simulink library "carnot"  (R2018b)
settings: Solver=VariableStepAuto  StartTime=0.0  StopTime=10.0  RelTol=1e-3
undefined symbols (not defined in the file or in its folder): A, A_earth, acol, Acol, ActPower1, ActPower2, ActPower3, Ad, Ad0, Ar, Au, Au0, Azimuth_Angle, B, Bd, Bd0, Br, Bu, Bu0, C, c1, c2, c3, c33, c4, c5, c6, CarnotCallbacks_Density, CarnotCallbacks_Enthalpy, CarnotCallbacks_Enthalpy2Temperature, CarnotCallbacks_Entropy, CarnotCallbacks_Evaporation_Enthalpy, CarnotCallbacks_GlobalMessageLevel, CarnotCallbacks_Grashof, CarnotCallbacks_Heat_Capacity, CarnotCallbacks_Kinematic_Viscosity, CarnotCallbacks_PMV_PPD, CarnotCallbacks_Prandtl, CarnotCallbacks_Saturation_Property, CarnotCallbacks_Saturation_Temperature, CarnotCallbacks_Saturation_Value_Water, CarnotCallbacks_Specific_Volume, CarnotCallbacks_Thermal_Conductivity, CarnotCallbacks_Vapour_Content, CarnotCallbacks_Vapour_Pressure, Cd, Cdl, Cr, Cu, Davies, Dd, DE_TRY2010_04_averageYear, delta_grd, density, DiameterLastPiece, dl, DPConstant, DPLinear, DPQuadratic, Dr ... (+59)
libraries: $bdroot x429, simulink x36, simulink_extras x12
(part 2 of 22)

== system carnot/Hydraulics ==
  Fan_Const : Subsystem  mask(Fan constant){Vdotmax=1000, dia=0.5, p0=101300, mix=0.01, Tini=20, UA=3, mcp=1000, e0=10, e1=10, e2=-1}
      mask prompts: Vdotmax "Vdotmax : volume flowrate in m³/h"; dia "diameter at in- and outlet [m]"; p0 "air pressure in Pa"; mix "kg of water per kg of dry air"; Tini "ambient and start temperature in °C"; UA "Thermal loss coefficient to ambient in W/K"; mcp "mcp: thermal capacity of the node in J/K"; e0 "e0: constant coefficient in W"; e1 "e1: linear coefficient in W*s/kg"; e2 "e2: quadratic coefficient in W*(s/kg)²"
      mask help:
      | Model of a fan for air ventilation systems. Volume flowrate is constant according to the parameter Vdotmax and the control signal:
      | Vdot = Vdotmax * Ctrl
      | Keep in mind that the flowrate in the THB is the massflowrate in kg/s whereas the parameters of the fan have different units.
      | mdot = Vdot/3600 * density(Tamb, air_pressure, FluidAir, kgH2O/kgAir)
      | Use the option "thermal node" if you want the pump to have thermal capacity and losses to ambient (or if you want to break an algebraic loop in the temperature signal).
      | Electric power is calculated Pel = e0 + e1*mdot + e2*mdot^2
      mask Help: web(fullfile(path_carnot('help'),'Fan_Const.html'),'-helpbrowser')
      mask TypeOptions dia: Pump_Const/dia
      mask TypeOptions mix: Pump_Const/mix
      mask TypeOptions Tini: Pump_Const/Tini
      mask TypeOptions UA: Pump_Const/UA
      mask TypeOptions mcp: Pump_Const/mcp
      mask TypeOptions e0: Pump_Const/e0
      mask TypeOptions e1: Pump_Const/e1
      mask TypeOptions e2: Pump_Const/e2
      mask DialogControl ParameterTabVar0 Prompt: Hydraulic
      mask DialogControl Container7 Prompt: Initial Values
      mask DialogControl ParameterTabVar012 Prompt: Thermal
      mask DialogControl ParameterTabVar01 Prompt: Electric
      mask Display:
      | plot(-40,-20,130,100, ...
      |     [0,0,10,30,50,70,80,80,70,50,30,10,0],[50,30,10,0,0,10,30,50,70,80,80,70,50], ...
      |     [80,10],[50,70], ...
      |     [80,10],[30,10])
  Flow_Diverter : Subsystem  mask(flow diverter, fixed rate){}
      mask help:
      | The block diverts an incoming massflow according to:
      | mdot1 = mdot * fdiv
      | mdot2 = mdot * (1-fdiv)
      | fdiv is limited to the range [0..1]
      mask Help: web(fullfile(path_carnot('help'),'Flow_Diverter.html'),'-helpbrowser')
      mask Display: plot(0,-5,120,65,[20 45 20 20],[20 30 40 20],[45 70 70 45],[30 20 40 30],[45 35 55 45],[30 10 10 30])
  Flow_Mixer : Subsystem  mask(flow mixer){}
      mask help:
      | Mixes two massflows. The new temperature is calculated by an energy balance. The output f_div may be fed back to the corresponding flow diverter upwards in flowdirection.
      | This model uses a Memory block to break an algebraic loop. Avoid using the variable-step solver ode15s or ode113 (see block help for details).
      mask Help: web(fullfile(path_carnot('help'),'Flow_Mixer.html'),'-helpbrowser')
      mask Display: plot(-25,-5,95,65,[20 45 20 20],[20 30 40 20],[45 70 70 45],[30 20 40 30],[45 35 55 45],[30 10 10 30])
  Flow_Mixer_Thermostatic : Subsystem  mask(thermostatic flow mixer){t=10}
      mask prompts: t "time constant for valve [s]"
      mask help:
      | The thermostatic flow mixer mixes cold and hot fluid to set a desired temperature and calculates the pressure drop.
      | Use together with flow_diverter_fixed_rate.
      mask init:
      | if t < 0.01
      |     t = 0.01;
      |     disp('Flow mixer thermostatic: time constant set to minimum value 0.01')
      | end
      | t1 = 1/t;
      mask Help: web(fullfile(path_carnot('help'),'Flow_Mixer.html'),'-helpbrowser')
      mask Display: plot(10,0,100,100,[40,60,60,40,40],[60,40,60,40,60],[44,50,56,44],[66,50,66,66],[50,50],[30,50],[56,44],[25,25],[50,50],[10,25])
  Mixing_Valve : Subsystem  mask(Mixing Valve){Art_A=equal percentage, Art_B=linear, kvs=1.6, psi_0=0.01, dt_V=30}
      mask prompts: Art_A "Valve characteristic A->AB"; Art_B "Valve characteristic B->AB"; kvs "Kvs: flow coefficient of the open valve in m³/h"; psi_0 "Psi_0: relative flow coefficient Kv/Kvs of the closed valve"; dt_V "Valve running time in s"
      mask help:
      | Mixes two massflows and calculates the pressure drop of the branches. The new temperature is calculated by an energy balance. The output f_div may be fed back to the corresponding flow diverter upwards in flowdirection.
      | This model uses a Memory block to break an algebraic loop. Avoid using the variable-step solver ode15s or ode113 (see block help for details).
      mask Help: web(fullfile(path_carnot('help'),'Mixing_Valve.html'),'-helpbrowser')
      mask TypeOptions Art_A: Valve_A/vtyp
      mask TypeOptions Art_B: Valve_B/vtyp
      mask TypeOptions kvs: Valve_A/kvs | Valve_B/kvs
      mask TypeOptions psi_0: Valve_A/psi_0 | Valve_B/psi_0
      mask TypeOptions dt_V: Valve_A/dt_V | Valve_B/dt_V
      mask Display:
      | plot(-20,-5,110,90,...
      |     [20 50 20 20],[20 30 40 20],...
      |     [50 80 80 50],[30 20 40 30],...
      |     [50 40 60 50],[30 10 10 30],...
      |     [50,50],[45,30],...
      |     [40,30,30,40,60,70,70,60,40],[45,50,60,65,65,60,50,45,45],...
      |     [60,60,50,40,40],[50,60,55,60,50])
  Pipe : Subsystem  mask(pipe){dia=0.02, len=10, hgt=5, uloss=100/20/10, cond=0, cwall=1000, t0=20, lin=100/0.2, qua=100/0.2^2, nodes=10}
      mask prompts: dia "diameter [m]"; len "length of pipe [m]"; hgt "static height [m], positive for outlet above"; uloss "heat losses per length [W/(m*K)]"; cond "effective conductivity in axial direction [W/(m*K)]"; cwall "capacity of pipewall per length in [J/(m*K)]"; t0 "initial temperature [degree Celsius]"; lin "pressure drop linear in massflow [Pa*s/kg]"; qua "pressure drop quadratic in massflow [Pa*s²/kg²]"; nodes "number of nodes"
      mask help:
      | Multinode pipe with capacity and simlified pressure drop calculation. The pressure drop is a quadratic function of the massflow. The dependance of the quadratic term on the Reynolds number is neglected. The flow is calculated by the upwind scheme heat conduction between nodes by central differences (Patankar 1980).
      | heat loss: ul = 2*Conductivity*pi*d_in*Length/Length/(d_in*ln(d_out/d_in))
      | The pressure change due to static height can usually be neglected for closes loop pumped systems.
      mask init:
      | if dia < 0.001
      |     dia = 0.001;
      |     disp('Warning in Pipe: diameter set to minimum value 0.001 m')
      | end
      | if len < 0.001
      |     len = 0.001;
      |     disp('Warning in Pipe: length set to minimum value 0.001 m')
      | end
      | if cwall < 0.001
      |     cwall = 0.001;
      |     disp('Warning in Pipe: heat capacity of the wall set to minimum value 0.001 m')
      | end
      | if nodes < 1
      |     nodes = 1;
      |     disp('Warning in Pipe: number of nodes set to minimum 1')
      | end
      mask Help: web(fullfile(path_carnot('help'),'Pipe.html'),'-helpbrowser')
      mask DialogControl ParameterTabVar0 Prompt: Geometry
      mask DialogControl ParameterTabVar01 Prompt: Thermal
      mask DialogControl ParameterTabVar012 Prompt: Hydraulic
      mask DialogControl ParameterTabVar0123 Prompt: Calculation
      mask Display: plot(0,0,100,100,[24,27,27,24,75,80,80,75,24,20,20,24],[60,53,46,40,40,46,55,60,60,53,46,40])
  Pipe_BiFlow : Subsystem  mask(Pipe Biflow){t0=20, hgt=1273.2395, stgtype=1, tini=[20 20 20 20 20 20 20 20 20 20], mpts=[1 2 3 4 5 6 7 8 9 10], PathName=fullfile(path_carnot('libsl'),'Hydraulics','Pipe_BiFlow','parameter_set'), FileName='PipeBF_set1.mat', userPath=off, userParam=off, uwall=1, ubot=0, utop=0, axcond=1, volume=10, dia=0.1, standing=standing cylinder, nodes=10, mpoints=10, pipe1inlet=1, pipe1outlet=0, pipe1dia=0.1, pipe2inlet=0, pipe2outlet=1, pipe2dia=0.1}
      mask prompts: t0 "Initial temperature (vector or scalar) in °C"; hgt "Length of pipe in m"; stgtype "Storage Type (0..5)"; tini "Start temperatures of nodes in °C"; mpts "Index to measured nodes"; PathName "Path"; FileName "Parameter set"; userPath "Edit path and name of parameter set"; userParam "User defined parameters"; uwall "Heat transfer coefficient to ambient [W/m²K]"; ubot "Heat transfer coefficient to ambient bottom [W/m²K]"; utop "Heat transfer coefficient to ambient top [W/m²K]"; axcond "Effective thermal conductivity [W/m/K]"; volume "Volume [m³]"; dia "Diameter [m]"; standing "Position"; nodes "Number of nodes"; mpoints "Number of node temperatures (for display)"; pipe1inlet "relative height of inlet, range from 0 (= bottom) to 1 (= top)"; pipe1outlet "relative height of outlet, range from 0 (= bottom) to 1 (= top)"; pipe1dia "Diameter of connection in m"; pipe2inlet "relative height of inlet, range from 0 (= bottom) to 1 (= top)"; pipe2outlet "relative height of outlet, range from 0 (= bottom) to 1 (= top)"; pipe2dia "Diameter of connection in m"
      mask help: Pipe model for flow in both directions. The model is based on a buffer storage tank but has no calculation for inversed thermocline.
      mask init:
      | [ok, param] = CarnotCallbacks_PipeBiflow('SetParam',1,gcbh,PathName,FileName);
      mask Help: web(fullfile(path_carnot('help'),'PipeBilfow.html'),'-helpbrowser')
      mask TypeOptions hgt: Pipe_Connection_1/hgt | Pipe_Connection_2/hgt
      mask TypeOptions stgtype: CreateSdat/stgtype
      mask TypeOptions tini: sfun_storageTnodes/tini
      mask TypeOptions mpts: select_T/Indices
      mask Callback userPath: [ok, param] = CarnotCallbacks_StorageConf('UserEdit',1,gcbh);
      mask Callback userParam: [ok, param] = CarnotCallbacks_StorageConf('UserEdit',1,gcbh);
      mask TypeOptions uwall: sfun_storageTnodes/uloss
      mask TypeOptions ubot: sfun_storageTnodes/ubot
      mask TypeOptions utop: sfun_storageTnodes/utop
      mask TypeOptions axcond: sfun_storageTnodes/cond
      mask TypeOptions volume: sfun_storageTnodes/volume | CreateSdat/volume
      mask TypeOptions dia: sfun_storageTnodes/dia | Pipe_Connection_1/dstg | Pipe_Connection_2/dstg
      mask TypeOptions standing: sfun_storageTnodes/standing
      mask TypeOptions nodes: sfun_storageTnodes/nodes | select_T/InputPortWidth | HX_EN12977_1/nodes | HX_EN12977_2/nodes | HX_EN12977_3/nodes | Pipe_Connection_1/nodes | Pipe_Connection_2/nodes | Pipe_Connection_3/nodes
      mask TypeOptions pipe1inlet: Pipe_Connection_1/h_in
      mask TypeOptions pipe1outlet: Pipe_Connection_1/h_out
      mask TypeOptions pipe1dia: Pipe_Connection_1/dpipe
      mask TypeOptions pipe2inlet: Pipe_Connection_2/h_in
      mask TypeOptions pipe2outlet: Pipe_Connection_2/h_out
      mask TypeOptions pipe2dia: Pipe_Connection_2/dpipe
      mask DialogControl Container14 Prompt: Infos
      mask DialogControl ParameterGroupVar Prompt: Picking a parameter set
      mask DialogControl Control3 Prompt: Carnot public data
      mask DialogControl Control3 Callback: [ok, file] = CarnotCallbacks_PipeBiflow('GetFilename',1,gcbh,'public');
      mask DialogControl Control4 Prompt: Carnot internal data
      mask DialogControl Control4 Callback: [ok, file] = CarnotCallbacks_PipeBiflow('GetFilename',1,gcbh,'internal');
      mask DialogControl Control2 Prompt: Selected path
      mask DialogControl Control2 Callback: [ok, file] = CarnotCallbacks_PipeBiflow('GetFilename',1,gcbh,'selected');
      mask DialogControl Container4 Prompt: Parameter values
      mask DialogControl Container6 Prompt: Pipe
      mask DialogControl Container8 Prompt: Connections
      mask DialogControl Container9 Prompt: Inlet 1
      mask DialogControl Container12 Prompt: Inlet 2
      mask DialogControl Control6 Prompt: Save in Carnot internal data
      mask DialogControl Control6 Callback: [ok, param] = CarnotCallbacks_PipeBiflow('SaveFilename',1,gcbh,'internal','PipeBF');
      mask DialogControl Control5 Prompt: Save in selected path
      mask DialogControl Control5 Callback: [ok, param] = CarnotCallbacks_PipeBiflow('SaveFilename',1,gcbh,'selected','PipeBF');
      mask Display:
      | % user defined picture file
      | picfile = fullfile(path_carnot('intlibsl'), 'Hydraulics','Pipe_Biflow', ...
      |     'parameter_set', 'Pipe_Biflow.jpg');
      | 
      | % show internal picture if defined
      | pic = false;
      | if  ~BlockIsInCarnotLibrary       % if not located in library
      |     if exist(picfile, 'file')
      |         image(imread(picfile), [0.25, 0, 0.45, 1])
      |         set_param(gcb, 'BackgroundColor', 'White')
      |         pic = true;
      |     end
      | end
      | 
      | % show public picture
      | if ~pic
      |     set_param(gcb, 'BackgroundColor', 'Red')
      |     plot(0,0,1,1,[24,27,27,24,75,80,80,75,24,20,20,24]/100,[60,53,46,40,40,46,55,60,60,53,46,40]/100)
      | end
  Pipe_Geometry : Subsystem  mask(Pipe Geometry){dia=0.02, len=10, hgt=10, uloss=100/20/10, cond=0, cwall=1000, t0=20, rough=0.04*1e-3, nbend=4, nodes=1}
      mask prompts: dia "diameter [m]"; len "length of pipe [m]"; hgt "static height [m], (positive for outlet above inlet)"; uloss "heat loss per length of pipe [W/(m*K)]"; cond "effective conductivity in the pipe [W/(m*K)]"; cwall "capacity of pipewall per length [J/(m*K)]"; t0 "initial temperature [degree centigrade]"; rough "roughness of pipe [m]"; nbend "number of 90° bends (45° = 0.667)"; nodes "number of nodes"
      mask help:
      | Multinode pipe with capacity and theoretical pressure drop calculation. The flow is calculated by the upwind scheme heat conduction between nodes by central differences (Patankar 1980).
      | heat loss: ul = 2*Conductivity*pi*d_in*Length/Length/(d_in*ln(d_out/d_in))
      | The pressure change due to static height can usually be neglected for closes loop pumped systems.
      mask init:
      | if dia < 0.001
      |     dia = 0.001;
      |     disp('Warning in Pipe: diameter set to minimum value 0.001 m')
      | end
      | if len < 0.001
      |     len = 0.001;
      |     disp('Warning in Pipe: length set to minimum value 0.001 m')
      | end
      | if cwall < 0.001
      |     cwall = 0.001;
      |     disp('Warning in Pipe: heat capacity of the wall set to minimum value 0.001 m')
      | end
      | if nodes < 1
      |     nodes = 1;
      |     disp('Warning in Pipe: number of nodes set to minimum 1')
      | end
      | if nbend < 0
      |     nbend = 0;
      |     disp('Warning in Pipe: number of bends set to minimum 0')
      | end
      | if rough < 0
      |     rough = 0;
      |     disp('Warning in Pipe: roughness of nodes set to minimum 0 m')
      | end
      mask Help: web(fullfile(path_carnot('help'),'Pipe_Geometry.html'),'-helpbrowser')
      mask DialogControl ParameterTabVar0 Prompt: Geometry
      mask DialogControl ParameterTabVar01 Prompt: Thermal
      mask DialogControl ParameterTabVar012 Prompt: Hydraulic
      mask DialogControl ParameterTabVar0123 Prompt: Calculation
      mask Display: plot(0,0,90,100,[8,12,16,16,12,8,8],[46,38,46,55,62,55,46],[12,33,48,52,70,73,73,70,50,35,30,12],[38,49,30,30,50,55,65,70,50,70,70,62])
  Pipe_Isolation : Subsystem  mask(pipe with relative isolation thickness){dia=0.02, len=10, hgt=0, isolat=43.72, condiso=0.05, cond=0, cwall=1000, t0=20, lin=100/0.2, qua=100/0.2^2, nodes=10}
      mask prompts: dia "Diameter [m]"; len "Length of pipe [m]"; hgt "difference in static height [m], positive for outlet above"; isolat "Isolation thickness in % (100%: isolation thickness = diameter, minimum 1%)"; condiso "Thermal conductivity of isolation [W/(m*K)]"; cond "Effective conductivity in the pipe [W/(m*K)]"; cwall "capacity of pipewall per length in [J/(m*K)]"; t0 "initial temperature [degree centigrade]"; lin "pressure drop linear in massflow [Pa*s/kg]"; qua "pressure drop quadratic in massflow [Pa*s²/kg²]"; nodes "number of nodes"
      mask help:
      | Multinode pipe with capacity and easy pressure drop calculation. The pressure drop is a quadratic function of the massflow. The dependance of the quadratic term on the Reynolds number is neglected. The flow is calculated by the upwind scheme heat conduction between nodes by central differences (Patankar 1980).
      | Isolation thickness in percent of the diameter. Heat loss:
      | ul = 2*conductivity*pi*d*Length/Length/(d*log(((2*percent+1)d)/d))
      | The pressure change due to static height can usually be neglected for closes loop pumped systems.
      mask init:
      | if dia < 0.001
      |     dia = 0.001;
      |     disp('Warning in Pipe: diameter set to minimum value 0.001 m')
      | end
      | if len < 0.001
      |     len = 0.001;
      |     disp('Warning in Pipe: length set to minimum value 0.001 m')
      | end
      | if cwall < 0.001
      |     cwall = 0.001;
      |     disp('Warning in Pipe: heat capacity of the wall set to minimum value 0.001 m')
      | end
      | if nodes < 1
      |     nodes = 1;
      |     disp('Warning in Pipe: number of nodes set to minimum 1')
      | end
      | if isolat < 1
      |     isolat = 1;
      |     disp('Warning in Pipe: Isolation set to minimum 1%')
      | end
      | uloss = 2*condiso*pi/(log(0.01*isolat*2+1));
      mask Help: web(fullfile(path_carnot('help'),'Pipe_Isolation.html'),'-helpbrowser')
      mask DialogControl ParameterTabVar0 Prompt: Geometry
      mask DialogControl ParameterTabVar01 Prompt: Thermal
      mask DialogControl ParameterTabVar012 Prompt: Hydraulic
      mask DialogControl ParameterTabVar0123 Prompt: Calculation
      mask Display: plot(-20,10,130,90,[0,2,5,7,5,2,0],[55,50,50,55,60,60,55],[96,99,100,99,96],[50,50,55,60,60],[10,13,17,19,19,17,13,10],[50,45,45,50,60,65,65,60],[5,15,17,17,15,5],[50,50,52,58,60,60],[17,93,96,96,92,17],[45,45,46,62,65,65])
  Pump_Additional : Subsystem  mask(Pump Additional){Tini=20, PathName=fullfile(path_carnot('libsl'), 'Hydraulics', 'Pump_Main', 'parameter_set'), FileName='Pump6m.mat', userPath=off, userParam=off, a0=60000, a1=-43200, a2=0, dia=0.025, UA=1, mcp=4182, e0=50, e1=28.8, e2=-10.368}
      mask prompts: Tini "Ambient temperature for losses and initial temperture in °C"; PathName "Path"; FileName "Parameter set"; userPath "Edit path and name of parameter set"; userParam "User defined parameters"; a0 "a0: pump head in [Pa] (pressure increase at zero flow)"; a1 "a1: pump characteristic linear coefficient [Pa*s/kg]"; a2 "a2: pump characteristic quadratic coefficient [Pa*(s/kg)²]"; dia "Diameter at in- and outlet [m]"; UA "UA: thermal loss coefficient in W/K"; mcp "mcp: thermal capacity of the node in J/K"; e0 "e0: constant coefficient in W"; e1 "e1: linear coefficient in W*s/kg"; e2 "e2: quadratic coefficient in W*(s/kg)²"
      mask help:
      | This is an additional pump in a circuit. Every circuit must have exactly ONE 'Pump_Main'. It may have several 'Pump_Additional' blocks. The pump adds dp_pump to the pressure drop of the circuit dp_circuit:
      |     dp_circuit = c + l*mdot + q*(mdot)²
      |     dp_pump_ = a0*Ctrl + a1*mdot +a2*(mdot)²
      |     dp_total = dp_pump - dp_circuit
      |     p1 = system_pressure + (a0*Ctrl - c) + (a1 - l) * mdot + (a2-q)*(mdot)²
      | with
      |   Ctrl : Control signal input [0..1]
      | Note: Pump_Additional uses the parameters sets as Pump_Main.
      mask init:
      | % callback to set parameters of model
      | [ok, param] = CarnotCallbacks_PumpAdditional('SetParameters',gcbh,PathName,FileName);
      mask Help: web(fullfile(path_carnot('help'),'Pump_Main.html'),'-helpbrowser')
      mask TypeOptions Tini: ThermalNodeTHB/Tini
      mask Callback userPath: [ok, param] = CarnotCallbacks_PumpAdditional('UserEdit',gcbh);
      mask Callback userParam: [ok, param] = CarnotCallbacks_PumpAdditional('UserEdit',gcbh);
      mask TypeOptions a0: PumpHead/Gain
      mask TypeOptions a1: PumpLinear/Value
      mask TypeOptions a2: PumpQuadratic/Value
      mask TypeOptions dia: dia/Value
      mask TypeOptions UA: ThermalNodeTHB/UA
      mask TypeOptions mcp: ThermalNodeTHB/mcp
      mask TypeOptions e0: ElectricConsumptionPump/e0
      mask TypeOptions e1: ElectricConsumptionPump/e1
      mask TypeOptions e2: ElectricConsumptionPump/e2
      mask DialogControl ParameterGroupFile Prompt: Picking a parameter set
      mask DialogControl Control1 Prompt: Carnot public data
      mask DialogControl Control1 Callback: [ok, file] = CarnotCallbacks_PumpAdditional('GetFilename',gcbh,'public');
      mask DialogControl Control3 Prompt: Carnot internal data
      mask DialogControl Control3 Callback: [ok, file] = CarnotCallbacks_PumpAdditional('GetFilename',gcbh,'internal');
      mask DialogControl Control4 Prompt: Selected path
      mask DialogControl Control4 Callback: [ok, file] = CarnotCallbacks_PumpAdditional('GetFilename',gcbh,'selected');
      mask DialogControl PrameterGroupUser Prompt: Parameter Values
      mask DialogControl Container9 Prompt: Hydraulic
      mask DialogControl Container7 Prompt: Thermal
      mask DialogControl Control9 Prompt: Thermal node for temperature:  mcp * dTnode/dt = UA*(Tamb-Tnode) + mdot*cp_in*(Tin-Tnode)
      mask DialogControl Container12 Prompt: Electric
      mask DialogControl Control7 Prompt: Power consumption  Pel = e0 + e1*mdot + e2*mdot²
      mask DialogControl Control5 Prompt: Save in Carnot internal data
      mask DialogControl Control5 Callback: [ok, param] = CarnotCallbacks_PumpAdditional('SaveFilename',gcbh,'internal','B');
      mask DialogControl Control6 Prompt: Save in selected path
      mask DialogControl Control6 Callback: [ok, param] = CarnotCallbacks_PumpAdditional('SaveFilename',gcbh,'selected','B');
      mask Display:
      | % user defined picture file
      | picfile = fullfile(path_carnot('intlibsl'), ...
      |         'Hydraulics', 'Pump_Additional', 'PumpAdditional.jpg');
      | 
      | pic = false;
      | if ~BlockIsInCarnotLibrary    % if not located in library any more
      |     if exist(picfile,'file') % show internal picture if defined
      |         image(imread(picfile), [0.2, 0, 0.6, 1])
      |         set_param(gcb, 'BackgroundColor', 'White')
      |         pic = true;
      |     end
      | end
      | if ~pic    % show public picture
      |     set_param(gcb, 'BackgroundColor', 'green')
      |     plot(0,0,1,1,[40,70,40,30,30,40,60,70,70,60,40]/100, ...
      |         [70,50,30,40,60,70,70,60,40,30,30]/100)
      |     disp('add')
      | end
  Pump_Const : Subsystem  mask(Pump constant){mdotmax=1200/3600, dia=0.02, p0=3e5, fluid_id=Water, mix=0, mix2=0, mix3=0, UA=3, mcp=4182, Tini=20, e0=10, e1=10, e2=-1}
      mask prompts: mdotmax "mdotmax : massflow rate in kg/s"; dia "diameter at in- and outlet [m]"; p0 "system pressure [Pa]"; fluid_id "fluid"; mix "percentage of fluid mix [0..1]"; mix2 "fluid mixture 2 [0..1]"; mix3 "fluid mixture 3 [0..1]"; UA "Thermal loss coefficient to ambient in W/K"; mcp "mcp: thermal capacity of the node in J/K"; Tini "Initial and ambient temperature in °C"; e0 "e0: constant coefficient in W"; e1 "e1: linear coefficient in W*s/kg"; e2 "e2: quadratic coefficient in W*(s/kg)²"
      mask help:
      | Set constant massflow rate according to the parameter mdotmax and the control signal:
      | mdot = mdotmax * Ctrl
      | Use the option "thermal node" if you want the pump to have thermal capacity and losses to ambient (or if you want to break an algebraic loop in the temperature signal).
      | Electric power is calculated Pel = e0 + e1*mdot + e2*mdot^2
      mask Help: web(fullfile(path_carnot('help'),'Pump_Const.html'),'-helpbrowser')
      mask TypeOptions mdotmax: Pump_basic/mdotmax
      mask TypeOptions dia: Pump_basic/dia
      mask TypeOptions p0: Pump_basic/p0
      mask TypeOptions fluid_id: Pump_basic/fluid_id
      mask TypeOptions mix: Pump_basic/mix
      mask TypeOptions mix2: Pump_basic/mix2
      mask TypeOptions mix3: Pump_basic/mix3
      mask TypeOptions UA: ThermalNodeTHB/UA
      mask TypeOptions mcp: ThermalNodeTHB/mcp
      mask TypeOptions Tini: ThermalNodeTHB/Tini
      mask TypeOptions e0: ElectricConsumptionPump/e0
      mask TypeOptions e1: ElectricConsumptionPump/e1
      mask TypeOptions e2: ElectricConsumptionPump/e2
      mask DialogControl ParameterTabVar0 Prompt: Hydraulic
      mask DialogControl ParameterTabVar012 Prompt: Thermal
      mask DialogControl ParameterTabVar01 Prompt: Electric
      mask Display:
      | plot(0,0,100,100,...
      |     [40,70,40,30,30,40,60,70,70,60,40],[70,50,30,40,60,70,70,60,40,30,30])
  Pump_Main : Subsystem  mask(Pump Main){Tini=20, p0=3e5, IDpreset=pressure drop, fluid=Water, mix=0, mix2=0, mix3=0, t1=1, PathName=fullfile(path_carnot('libsl'), 'Hydraulics', 'Pump_Main', 'parameter_set'), FileName='Pump6m.mat', userPath=off, userParam=off, a0=60000, a1=-43200, a2=0, dia=0.025, UA=1, mcp=4182, e0=50, e1=28.8, e2=-10.368}
      mask prompts: Tini "Ambient temperature for losses and initial temperture in °C"; p0 "System pressure at pump inlet [Pa]"; IDpreset "Pressure calculation"; mix "Fluid mixture    [0..1]"; mix2 "Fluid mixture 2 [0..1]"; mix3 "Fluid mixture 3 [0..1]"; t1 "Time constant [s] of PT1 transfer function for massflow"; PathName "Path"; FileName "Parameter set"; userPath "Edit path and name of parameter set"; userParam "User defined parameters"; a0 "a0: pump head in [Pa] (pressure increase at zero flow)"; a1 "a1: pump characteristic linear coefficient [Pa*s/kg]"; a2 "a2: pump characteristic quadratic coefficient [Pa*(s/kg)²]"; dia "Diameter at in- and outlet [m]"; UA "UA: thermal loss coefficient in W/K"; mcp "mcp: thermal capacity of the node in J/K"; e0 "e0: constant coefficient in W"; e1 "e1: linear coefficient in W*s/kg"; e2 "e2: quadratic coefficient in W*(s/kg)²"
      mask help:
      | This is the main pump in a circuit. Every circuit must have exactly ONE 'Pump_Main'. Use the 'Pump_Additional' blocks if you want to use more pumps.
      | The Pump_Main calculate massflow by setting pressure drop in the circuit (dp_circuit) equal to the pressure increase of the pump (dp_pump).
      |   dp_circuit = c + l*mdot + q*mdot²
      |   dp_pump_ = a0*Ctrl + a1*mdot +a2*mdot²
      | with
      |   mdot : massflow in kg/s
      |   Ctrl : Control signal input [0..1]
      mask init:
      | % callback to set parameters of model
      | [ok, param] = CarnotCallbacks_PumpMain('SetParameters',gcbh,PathName,FileName);
      mask Help: web(fullfile(path_carnot('help'),'Pump_Main.html'),'-helpbrowser')
      mask TypeOptions Tini: ThermalNodeTHB/Tini
      mask TypeOptions p0: basic_THB/p
      mask TypeOptions IDpreset: ID/IDpreset
      mask TypeOptions fluid: basic_THB/fluid
      mask TypeOptions mix: basic_THB/mix
      mask TypeOptions mix2: basic_THB/mix2
      mask TypeOptions mix3: basic_THB/mix3
      mask TypeOptions t1: Transfer Fcn/t1
      mask Callback userPath: [ok, param] = CarnotCallbacks_PumpMain('UserEdit',gcbh);
      mask Callback userParam: [ok, param] = CarnotCallbacks_PumpMain('UserEdit',gcbh);
      mask TypeOptions a0: PumpHead/Gain
      mask TypeOptions a1: PumpLinear/Value
      mask TypeOptions a2: PumpQuadratic/Value
      mask TypeOptions dia: basic_THB/dia
      mask TypeOptions UA: ThermalNodeTHB/UA
      mask TypeOptions mcp: ThermalNodeTHB/mcp
      mask TypeOptions e0: ElectricConsumptionPump/e0
      mask TypeOptions e1: ElectricConsumptionPump/e1
      mask TypeOptions e2: ElectricConsumptionPump/e2
      mask DialogControl ParameterGroupFile Prompt: Picking a parameter set
      mask DialogControl Control1 Prompt: Carnot public data
      mask DialogControl Control1 Callback: [ok, file] = CarnotCallbacks_PumpMain('GetFilename',gcbh,'public');
      mask DialogControl Control3 Prompt: Carnot internal data
      mask DialogControl Control3 Callback: [ok, file] = CarnotCallbacks_PumpMain('GetFilename',gcbh,'internal');
      mask DialogControl Control4 Prompt: Selected path
      mask DialogControl Control4 Callback: [ok, file] = CarnotCallbacks_PumpMain('GetFilename',gcbh,'selected');
      mask DialogControl PrameterGroupUser Prompt: Parameter Values
      mask DialogControl Container9 Prompt: Hydraulic
      mask DialogControl Container7 Prompt: Thermal
      mask DialogControl Control9 Prompt: Thermal node for temperature:  mcp * dTnode/dt = UA*(Tamb-Tnode) + mdot*cp_in*(Tin-Tnode)
      mask DialogControl Container14 Prompt: Electric
      mask DialogControl Control7 Prompt: Power consumption  Pel = e0 + e1*mdot + e2*mdot²
      mask DialogControl Control5 Prompt: Save in Carnot internal data
      mask DialogControl Control5 Callback: [ok, param] = CarnotCallbacks_PumpMain('SaveFilename',gcbh,'internal','B');
      mask DialogControl Control6 Prompt: Save in selected path
      mask DialogControl Control6 Callback: [ok, param] = CarnotCallbacks_PumpMain('SaveFilename',gcbh,'selected','B');
      mask Display:
      | % user defined picture file
      | picfile = fullfile(path_carnot('intlibsl'), ...
      |         'Hydraulics', 'Pump_Main', 'PumpMain.jpg');
      | 
      | pic = false;
      | if ~BlockIsInCarnotLibrary    % if not located in library any more
      |     if exist(picfile,'file') % show internal picture if defined
      |         image(imread(picfile), [0.2, 0, 0.6, 1])
      |         set_param(gcb, 'BackgroundColor', 'White')
      |         pic = true;
      |     end
      | end
      | if ~pic    % show public picture
      |     set_param(gcb, 'BackgroundColor', 'green')
      |     plot(0,0,1,1,[40,70,40,30,30,40,60,70,70,60,40]/100, ...
      |         [70,50,30,40,60,70,70,60,40,30,30]/100)
      |     disp('main')
      | end
  Pump_basic : Subsystem  mask(basic Pump){mdotmax=0.1, fluid_id=Water, mix=0, mix2=0, mix3=0, p0=3e5, dia=0.02, ID=No Pressure Drop, hgt=0}
      mask prompts: mdotmax "massflow rate [kg/s]"; fluid_id "fluid"; mix "percentage of fluid mix [0..1]"; mix2 "fluid mixture 2 [0..1]"; mix3 "fluid mixture 3 [0..1]"; p0 "system pressure [Pa]"; dia "diameter at in- and outlet [m]"; ID "ID (pressure drop calculation mode)"; hgt "static height in m (positive value above ground)"
      mask help:
      | Set constant massflow rate according to the control signal.
      | ID for pressure drop calculation:
      |     1    .. 9999 No Pressure Drop
      |     10001..19999 Pressure Drop from Massflow
      |     20001..inf   Full Pressure Drop with Static Height
      mask init:
      | mix = min(1, max(0, mix));
      | dia = max(0.001, dia);
      mask Help: web(fullfile(path_carnot('help'),'Pump_basic.html'),'-helpbrowser')
      mask TypeOptions mdotmax: mdot/Gain
      mask TypeOptions fluid_id: basic_THB/fluid
      mask TypeOptions mix: basic_THB/mix
      mask TypeOptions mix2: basic_THB/mix2
      mask TypeOptions mix3: basic_THB/mix3
      mask TypeOptions p0: basic_THB/p
      mask TypeOptions dia: basic_THB/dia
      mask TypeOptions ID: basic_THB/ID
      mask TypeOptions hgt: basic_THB/hgt
      mask Display:
      | plot(0,0,100,100, ...
      |     [40,70,40,30,30,40,60,70,70,60,40],[70,50,30,40,60,70,70,60,40,30,30])
  Thermosyphon : Subsystem  mask(thermosyphon){p0=3e5, dia=0.025, fluid_id=Water, mix=0, mix2=0, mix3=0, t1=1}
      mask prompts: p0 "static system pressure [Pa]"; dia "Diameter at in- and outlet [m]"; fluid_id "fluid"; mix "fluid mixture [0..1]"; mix2 "fluid mixture 2 [0..1]"; mix3 "fluid mixture 3 [0..1]"; t1 "Time constant of PT1 transfer function for massflow in s"
      mask help:
      | This block is a model of a "thermosyphon pump". Place it in natural convection systems as you would place a pump.
      | Assure that the sum of heights is zero. Otherwise the simulation will not start.
      | You may check the sum of heights by verifying the "Geodetic Height" in the THB at the inport of this block.
      | If the sum is not zero, the difference is displayed in the subsystem "Stop Simulation".
      | This model uses a Memory block to break an algebraic loop. Avoid using the variable-step solver ode15s or ode113 (see block help for details).
      | A unit delay block with a sample time ("time constant of the pump") limits the maximum stepsize.
      mask Help: web(fullfile(path_carnot('help'),'Thermosyphon.html'),'-helpbrowser')
      mask TypeOptions p0: basic_THB/p
      mask TypeOptions dia: basic_THB/dia
      mask TypeOptions fluid_id: basic_THB/fluid
      mask TypeOptions mix: basic_THB/mix
      mask TypeOptions mix2: basic_THB/mix2
      mask TypeOptions mix3: basic_THB/mix3
      mask TypeOptions t1: Transfer Fcn/t1
      mask DialogControl Container4 Prompt: Hydraulic
      mask Display: plot(0,0,100,100,[90,10],[80,90],[90,10],[70,80],[90,10],[20,10],[90,10],[30,20],[40,60,40,40],[60,50,40,60])
  Valve : Subsystem  mask(Valve Function){vtyp=linear, psi_0=0.04, kvs=1.6, dt_V=30}
      mask prompts: vtyp "Valve characteristic"; psi_0 "Psi_0: relative flow coefficient Kv/Kvs of the closed valve"; kvs "Kvs: flow coefficient of the open valve in m³/h"; dt_V "Valve running time in s"
      mask help:
      | Model of a valve with flow coefficient characteristic:
      | Linear                     psi = psi_0 + (1-psi_0)*h
      | Equal percentage    psi = psi_0 * (1/psi_0)^h)
      | with
      |   h = H/H100   relative opening
      |   Kv                 flow coefficient in m³/h
      |   Kv = Vdot * sqrt(1e5Pa/dp * density/1000kg/m³)
      |   Kvs                flow coefficient  in m³/h of the fully opened valve.
      |   psi = Kv/Kvs  relative flow coefficient
      |   Vdot             volumetric flow rate in m³/h
      | Typical value for the relative flow coefficient at zero opening psi_0 is 0.04
      mask Help: web(fullfile(path_carnot('help'),'Valve.html'),'-helpbrowser')
      mask TypeOptions vtyp: relFlowCoefficientFunction/vtyp
      mask TypeOptions psi_0: relFlowCoefficientFunction/psi_0
      mask TypeOptions kvs: relFlowCoeff2qua/kvs
      mask TypeOptions dt_V: Rate Limiter/dt_V
      mask Display:
      | plot(-30,-20,130,120,[10,90,90,10,10],[50,0,50,0,50],...
      |     [50,50],[50,25],...
      |     [40,30,30,40,60,70,70,60,40],[50,60,80,90,90,80,60,50,50],...
      |     [60,60,50,40,40],[60,80,70,80,60])
  Valve_Thermostatic : Subsystem  mask(thermostatic valve){p=4, op=0.5, bl=0.2, ts=1, dt_V=1, ART=linear, kvs=2, psi_0=0.04}
      mask prompts: p "Proportional range in K"; op "Operation point (valve position at set temperature)"; bl "Hysteresis or play in K"; ts "First order hold for temperature sensor in s"; dt_V "Valve running time in s"; ART "Valve characteristic"; kvs "Kvs: flow coefficient of the open valve in m³/h"; psi_0 "Psi_0: relative flow coefficient Kv/Kvs of the closed valve"
      mask help: Thermostatic valve for a radiator.
      mask Help: web(fullfile(path_carnot('help'),'Valve_Thermostatic.html'),'-helpbrowser')
      mask TypeOptions p: Thermostat_Proportional/p
      mask TypeOptions op: Thermostat_Proportional/op
      mask TypeOptions bl: Thermostat_Proportional/bl
      mask TypeOptions ts: Thermostat_Proportional/ts
      mask TypeOptions dt_V: Valve/dt_V
      mask TypeOptions ART: Valve/vtyp
      mask TypeOptions kvs: Valve/kvs
      mask TypeOptions psi_0: Valve/psi_0
      mask DialogControl ParameterTabVar0 Prompt: Thermostat
      mask DialogControl ParameterTabVar01 Prompt: Hydraulic
      mask Display:
      | plot(-20,-20,120,120,[10,90,90,10,10],[50,0,50,0,50],...
      |     [50,50],[50,25],...
      |     [40,30,30,40,60,70,70,60,40],[50,60,80,90,90,80,60,50,50],...
      |     [60,40],[80,80],[50,50],[60,80])
  Valve_table : Subsystem  mask(Valve Function){h=[0 1], psi=[0.04 1], kvs=0.9, dt_V=0.01}
      mask prompts: h "Ctrl: relative valve position data (vector)"; psi "Psi: relative flow coefficient data - vector of length(Ctrl)"; kvs "Kvs: flow coefficient of the open valve in m³/h"; dt_V "Valve running time in s"
      mask help:
      | Model of a valve with a lookup table for the flow coefficient characteristic:
      |   psi = lookuptable(h)
      | with
      |   h = H/H100   relative opening
      |   Kv                 flow coefficient in m³/h
      |   Kv = Vdot * sqrt(1e5Pa/dp * density/1000kg/m³)
      |   Kvs                flow coefficient  in m³/h of the fully opened valve.
      |   psi = Kv/Kvs  relative flow coefficient
      |   Vdot             volumetric flow rate in m³/h
      | Note: Psi must be > 0 for Ctrl = 0
      | Typical value for the relative flow coefficient at zero opening psi_0 is 0.04
      mask Help: web(fullfile(path_carnot('help'),'Valve_table.html'),'-helpbrowser')
      mask TypeOptions h: h2psi_table/BreakpointsForDimension1
      mask TypeOptions psi: h2psi_table/Table
      mask TypeOptions kvs: relFlowCoeff2qua/kvs
      mask TypeOptions dt_V: Rate Limiter/dt_V
      mask Display:
      | plot(-30,-20,130,120,[10,90,90,10,10],[50,0,50,0,50],...
      |     [50,50],[50,25],...
      |     [40,30,30,40,60,70,70,60,40],[50,60,80,90,90,80,60,50,50],...
      |     [60,60,50,40,40],[60,80,70,80,60])

== system carnot/License ==
  note: This file is part of the CARNOT Blockset.
      |  	Copyright (c) 1998-2022, Solar-Institute Juelich of the FH Aachen.
      |  	Additional Copyright for file and models see list auf authors.
      |  	All rights reserved.
      |  	Redistribution and use in source and binary forms, with or without
      |  	modification, are permitted provided that the following conditions are met:
      |  	1. Redistributions of source code must retain the above copyright notice,
      |  	   this list of conditions and the following disclaimer.
      |  	2. Redistributions in binary form must reproduce the above copyright
      |  	   notice, this list of conditions and the following disclaimer in the
      |  	   documentation and/or other materials provided with the distribution.
      |  	3. Neither the name of the copyright holder nor the names of its
      |   	   contributors may be used to endorse or promote products derived from
      |   	   this software without specific prior written permission.
      |
      |  THIS SOFTWARE IS PROVIDED BY THE COPYRIGHT HOLDERS AND CONTRIBUTORS "AS IS"
      |  	AND ANY EXPRESS OR IMPLIED WARRANTIES, INCLUDING, BUT NOT LIMITED TO, THE
      |  	IMPLIED WARRANTIES OF MERCHANTABILITY AND FITNESS FOR A PARTICULAR PURPOSE
      |  	ARE DISCLAIMED. IN NO EVENT SHALL THE COPYRIGHT HOLDER OR CONTRIBUTORS BE
      |  	LIABLE FOR ANY DIRECT, INDIRECT, INCIDENTAL, SPECIAL, EXEMPLARY, OR
      |  	CONSEQUENTIAL DAMAGES (INCLUDING, BUT NOT LIMITED TO, PROCUREMENT OF
      |  	SUBSTITUTE GOODS OR SERVICES; LOSS OF USE, DATA, OR PROFITS; OR BUSINESS
      |  	INTERRUPTION) HOWEVER CAUSED AND ON ANY THEORY OF LIABILITY, WHETHER IN
      |  	CONTRACT, STRICT LIABILITY, OR TORT (INCLUDING NEGLIGENCE OR OTHERWISE)
      |  	ARISING IN ANY WAY OUT OF THE USE OF THIS SOFTWARE, EVEN IF ADVISED OF
      |  	THE POSSIBILITY OF SUCH DAMAGE.

== system carnot/Load ==
  General : Subsystem
      mask Display: plot(0,0,100,100,[100,0,0],[-0,-0,100],[100,95,81,72,62,54,51,36,26,20,17,15,13,10,0],[10,46,32,57,96,96,31,39,5,1,87,33,47,50,10])
  Hot_Water_Tapping : Subsystem
      mask Display: plot(0,0,100,100,[44,67,67,45,45,40,40,44],[80,80,72,72,60,60,76,80],[60,45],[90,90],[53,53],[80,90],[24,29,70,75,24],[30,10,10,30,30],[42,42],[32,58],[46,44],[34,54],[38,40],[34,56])
  Houses : Subsystem
      mask Display: plot(0,0,80,90,[30,30,60,60,30],[20,50,50,20,20],[47,47,56,56,47],[40,30,30,40,40],[42,42,34,34],[20,40,40,20],[62,45,28],[48,70,48])
